simulink model "Transient_Diffussion"  (R2021b)
settings: Solver=VariableStepAuto  StartTime=0.0  StopTime=10.0  RelTol=1e-3
undefined symbols (not defined in the file or in its folder): Co, Cs, Cx, D, Do, ferror, Qd, T, x, Zvalue
settings Model: Creator=lucio  LastModifiedBy=lucio
settings DataIOCC: ReturnWorkspaceOutputs=off

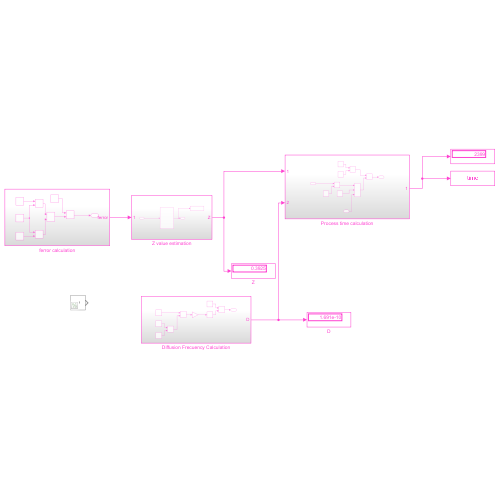
[thumbnail: Simulink's stored preview of the top-level diagram]
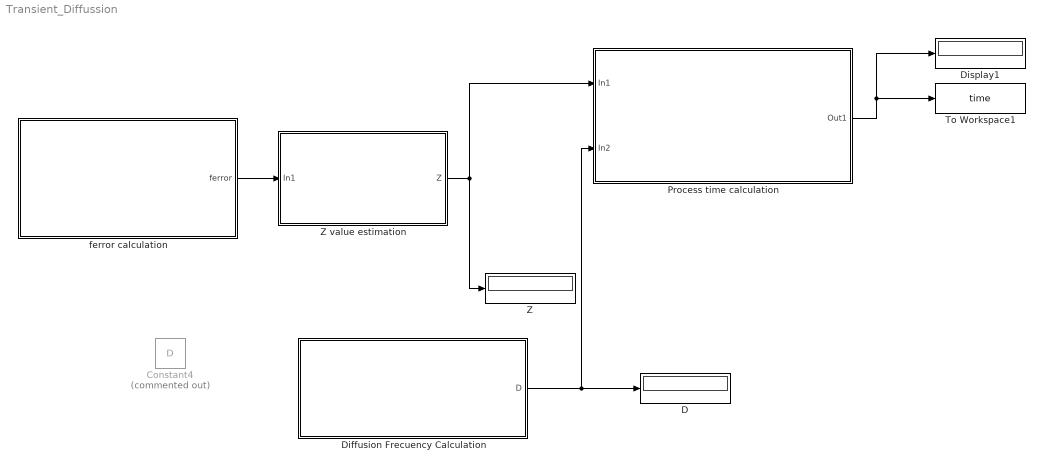
== system Transient_Diffussion ==
  Constant4 : Constant  Commented=on  Value=D
  D : Display
  Diffusion Frecuency Calculation : Subsystem
  Display1 : Display
  Process time calculation : Subsystem
  To Workspace1 : ToWorkspace  VariableName=time  SampleTime=-1
  Z : Display
  Z value estimation : Subsystem
  ferror calculation : Subsystem
  wires:
  Diffusion Frecuency Calculation/1(D) -> D/1, Process time calculation/2(In2)
  Z value estimation/1(Z) -> Process time calculation/1(In1), Z/1
  ferror calculation/1(ferror) -> Z value estimation/1(In1)
  Process time calculation/1(Out1) -> Display1/1, To Workspace1/1

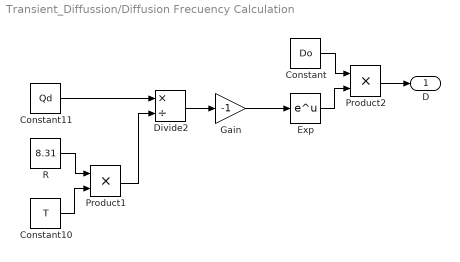
== system Transient_Diffussion/Diffusion Frecuency Calculation ==
  Constant : Constant  Value=Do
  Constant10 : Constant  Value=T
  Constant11 : Constant  Value=Qd
  Divide2 : Product  Inputs=*/
  Exp : Math  SaturateOnIntegerOverflow=on
  Gain : Gain  Gain=-1
  Product1 : Product
  Product2 : Product
  R : Constant  Value=8.31
  D : Outport
  wires:
  Constant/1 -> Product2/1
  Gain/1 -> Exp/1
  R/1 -> Product1/1
  Constant10/1 -> Product1/2
  Constant11/1 -> Divide2/1
  Product1/1 -> Divide2/2
  Divide2/1 -> Gain/1
  Exp/1 -> Product2/2
  Product2/1 -> D/1

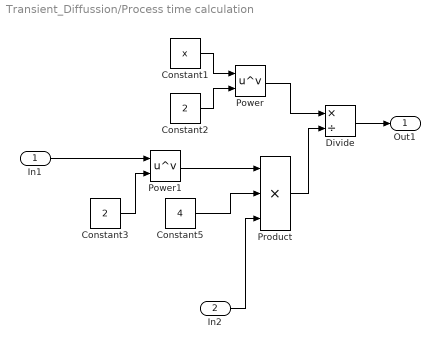
== system Transient_Diffussion/Process time calculation ==
  In1 : Inport
  In2 : Inport  Port=2
  Constant1 : Constant  Value=x
  Constant2 : Constant  Value=2
  Constant3 : Constant  Value=2
  Constant5 : Constant  Value=4
  Divide : Product  Inputs=*/
  Power : Math  Operator=pow  SaturateOnIntegerOverflow=on
  Power1 : Math  Operator=pow  SaturateOnIntegerOverflow=on
  Product : Product  Inputs=3
  Out1 : Outport
  wires:
  Constant2/1 -> Power/2
  Power1/1 -> Product/1
  Constant1/1 -> Power/1
  In1/1 -> Power1/1
  Product/1 -> Divide/2
  Constant3/1 -> Power1/2
  Constant5/1 -> Product/2
  Power/1 -> Divide/1
  Divide/1 -> Out1/1
  In2/1 -> Product/3

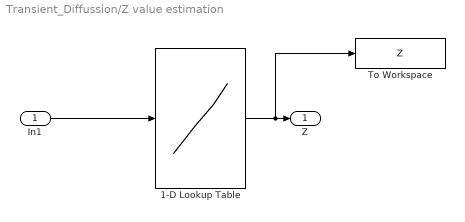
== system Transient_Diffussion/Z value estimation ==
  In1 : Inport
  1-D Lookup Table : Lookup_n-D  NumberOfTableDimensions=1  BreakpointsForDimension1=ferror  Table=Zvalue  InternalRulePriority=Speed  RndMeth=Simplest  InputSameDT=on
  To Workspace : ToWorkspace  VariableName=Z  SampleTime=-1
  Z : Outport
  wires:
  1-D Lookup Table/1 -> To Workspace/1, Z/1
  In1/1 -> 1-D Lookup Table/1

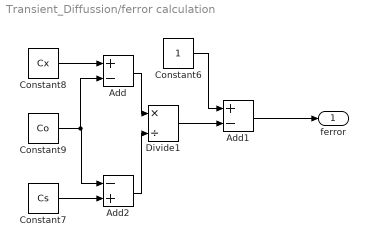
== system Transient_Diffussion/ferror calculation ==
  Add : Sum  Inputs=+-
  Add1 : Sum  Inputs=+-
  Add2 : Sum  Inputs=-+
  Constant6 : Constant
  Constant7 : Constant  Value=Cs
  Constant8 : Constant  Value=Cx
  Constant9 : Constant  Value=Co
  Divide1 : Product  Inputs=*/
  ferror : Outport
  wires:
  Constant8/1 -> Add/1
  Constant6/1 -> Add1/1
  Divide1/1 -> Add1/2
  Constant9/1 -> Add/2, Add2/1
  Add2/1 -> Divide1/2
  Constant7/1 -> Add2/2
  Add/1 -> Divide1/1
  Add1/1 -> ferror/1
